simulink model "prova_SMC"  (R2025b)
settings: Solver=VariableStepAuto  StartTime=0.0  StopTime=10.0  RelTol=1e-3
settings Model: Creator=lucag  LastModifiedBy=lucag

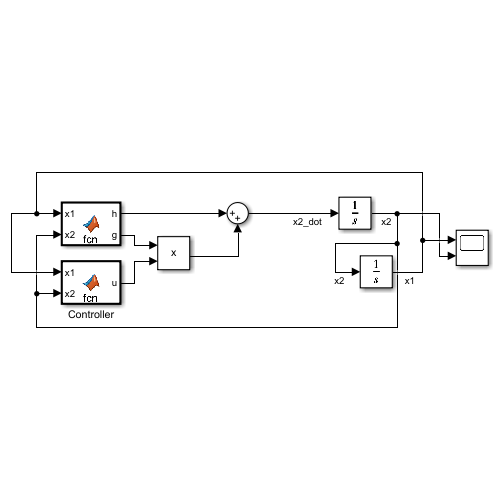
[thumbnail: Simulink's stored preview of the top-level diagram]
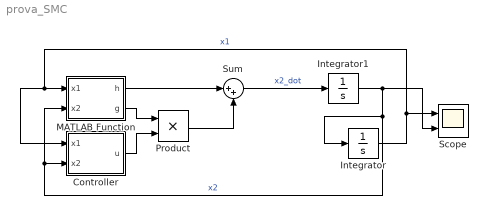
== system prova_SMC ==
  Controller : MATLAB Function  TreatAsAtomicUnit=on
  Integrator : Integrator  InitialCondition=3
  Integrator1 : Integrator  InitialCondition=5
  MATLAB Function : MATLAB Function  TreatAsAtomicUnit=on
  Product : Product
  Scope : Scope  NumInputPorts=2
      settings: ActiveDisplayYMinimum=-32.409202047646254  ActiveDisplayYMaximum=9.1565780052940262
  Sum : Sum  Inputs=|++
  wires:
  Integrator1/1 -> Controller/2(x2), MATLAB Function/2(x2), Integrator/1, Scope/2  "x2"
  Controller/1(u) -> Product/2
  MATLAB Function/2(g) -> Product/1
  MATLAB Function/1(h) -> Sum/1
  Product/1 -> Sum/2
  Sum/1 -> Integrator1/1  "x2_dot"
  Integrator/1 -> Scope/1, MATLAB Function/1(x1), Controller/1(x1)  "x1"

== matlab function prova_SMC/MATLAB Function ==
  data: x1 input; h output; x2 input; g output
function [h,g] = fcn(x1, x2)
    h = sin(x1+x2);
    g = 1 + 0.1*x2^2;
end

== matlab function prova_SMC/Controller ==
  data: x1 input; u output; x2 input
function u = fcn(x1, x2)
    k = 10;
    a = 2;
    u = -k*sign(x2+a*x1);
end
